simulink subsystem "IMU_6DOF"  (R2023a)
settings: Solver=VariableStepAuto  StartTime=0.0  StopTime=10.0  RelTol=1e-3
undefined symbols (not defined in the file): ODR
libraries: mbedblockslib x1
settings Model: Creator=JesseJabezArendse  LastModifiedBy=JesseJabezArendse

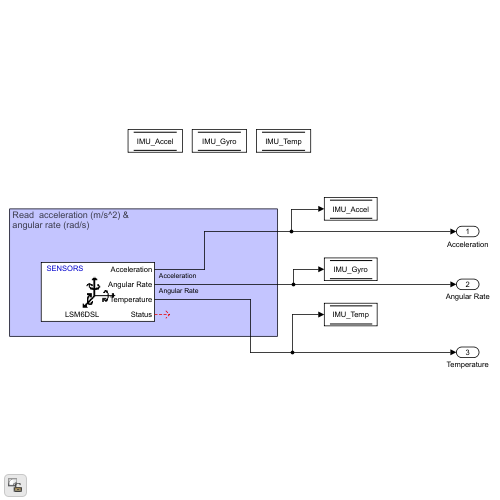
[thumbnail: Simulink's stored preview of the top-level diagram]
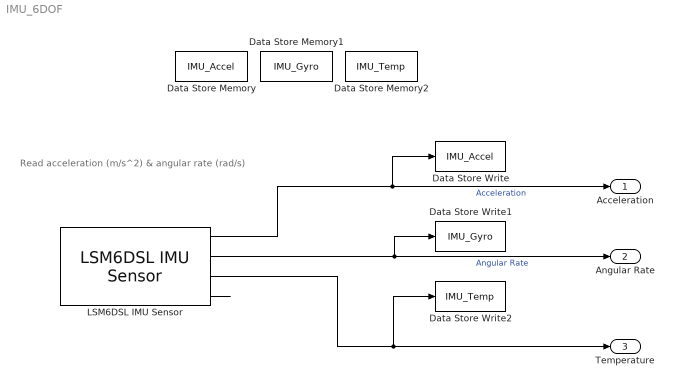
== system IMU_6DOF ==
  note: Read  acceleration (m/s^2) &
      | angular rate (rad/s)
  Data Store Memory : DataStoreMemory  DataStoreName=IMU_Accel  WriteAfterWriteMsg=warning  ShowAdditionalParam=off  OutDataTypeStr=double  Dimensions=3
  Data Store Memory1 : DataStoreMemory  DataStoreName=IMU_Gyro  WriteAfterWriteMsg=warning  ShowAdditionalParam=off  OutDataTypeStr=double  Dimensions=3
  Data Store Memory2 : DataStoreMemory  DataStoreName=IMU_Temp  WriteAfterWriteMsg=warning  ShowAdditionalParam=off  OutDataTypeStr=double  Dimensions=1
  Data Store Write : DataStoreWrite  DataStoreName=IMU_Accel  IndexOptions=Index vector (dialog)  Indices=1  OutputSizes=1
  Data Store Write1 : DataStoreWrite  DataStoreName=IMU_Gyro  IndexOptions=Index vector (dialog)  Indices=1  OutputSizes=1
  Data Store Write2 : DataStoreWrite  DataStoreName=IMU_Temp  IndexOptions=Index vector (dialog)  Indices=1  OutputSizes=1
  LSM6DSL IMU Sensor : mbedblockslib/LSM6DSL IMU Sensor  I2CModule=0  I2CAddress=0x6B  IsActiveAcceleration=on  IsActiveAngularRate=on  IsActiveTemperature=on  IsActiveStatus=on  IsActiveTimeStamp=off  SampleTime=0.01  QueueSizeFactor=3  AccelerometerRange=+/- 4g  AccelerometerODR=104 Hz  AccelLPF1BW=ODR/2  AccelSelectCompositeFilter=No filter  AccelLPF2BW=ODR/50  AccelHPFBW=ODR/100  GyroscopeRange=250 dps  GyroscopeODR=104 Hz  EnableGyroHPF=off  GyroHPFBW=0.016 Hz  EnableGyroLPF=off  GyroLPFBWMode=0
      settings: LibrarySourceBlock=stmnucleosensorslib/LSM6DSL IMU Sensor
  Acceleration : Outport
  Angular Rate : Outport  Port=2
  Temperature : Outport  Port=3
  wires:
  LSM6DSL IMU Sensor/1 -> Acceleration/1, Data Store Write/1  "Acceleration"
  LSM6DSL IMU Sensor/2 -> Angular Rate/1, Data Store Write1/1  "Angular Rate"
  LSM6DSL IMU Sensor/3 -> Temperature/1, Data Store Write2/1
  LSM6DSL IMU Sensor/4 -> ?
